simulink model "3DoFManipulatorWithBLDCM_SIMULATION"  (R2023b)
settings: Solver=VariableStepAuto  StartTime=0.0  StopTime=10  MaxStep=1e-4  RelTol=1e-3
undefined symbols (not defined in the file): X, Y, Z
libraries: spsMosfetLib x18, sm_lib x11, nesl_utility x7, eeGeneralControl x6, spsDCVoltageSourceLib x3, spsGroundLib x3, spsThreePhaseSeriesRLCBranchLib x3, spsThreePhaseVIMeasurementLib x3, slpidlib x3, sps_lib x1
(part 3 of 3)

== matlab function 3DoFManipulatorWithBLDCM_SIMULATION/BLDC/Actuator Link1/Three Phase Inverter/MOTOR_SPEED_BLOCK1 ==
  data: U_U input; U_V input; U_W input; U_U_PWM output; PWM input; U_V_PWM output; U_W_PWM output
function [U_U_PWM, U_V_PWM, U_W_PWM] = PWM_SPEED_BLOCK(U_U, U_V, U_W, PWM)
%#codegen

%    This function was generated by the Symbolic Math Toolbox version 23.2.
%    20-Mar-2024 19:58:52

U_U_PWM = 0;
U_V_PWM = 0;
U_W_PWM = 0;

% Apply PWM scaling based on input and PWM signal
if U_U ~= 0 && PWM ~= 0
    U_U_PWM = U_U * PWM;
end
if U_V ~= 0 && PWM ~= 0
    U_V_PWM = U_V * PWM;
end
if U_W ~= 0 && PWM ~= 0
    U_W_PWM = U_W * PWM;
end

end

== matlab function 3DoFManipulatorWithBLDCM_SIMULATION/BLDC/Actuator Link2/Three Phase Inverter/MOTOR_SPEED_BLOCK1 ==
  data: U_U input; U_V input; U_W input; U_U_PWM output; PWM input; U_V_PWM output; U_W_PWM output
function [U_U_PWM, U_V_PWM, U_W_PWM] = PWM_SPEED_BLOCK(U_U, U_V, U_W, PWM)
%#codegen

%    This function was generated by the Symbolic Math Toolbox version 23.2.
%    20-Mar-2024 19:58:52

U_U_PWM = 0;
U_V_PWM = 0;
U_W_PWM = 0;

% Apply PWM scaling based on input and PWM signal
if U_U ~= 0 && PWM ~= 0
    U_U_PWM = U_U * PWM;
end
if U_V ~= 0 && PWM ~= 0
    U_V_PWM = U_V * PWM;
end
if U_W ~= 0 && PWM ~= 0
    U_W_PWM = U_W * PWM;
end

end

== matlab function 3DoFManipulatorWithBLDCM_SIMULATION/Feedforward Control/PWM LINK1/MOTOR_SPEED_BLOCK3 ==
  data: e_diff input; dC output; p output
function [dC, p] = PWM_SPEED_BLOCK(e_diff)
%#codegen

%    This function was generated by the Symbolic Math Toolbox version 23.2.
%    20-Mar-2024 19:58:52

p = 0.0001;
p = max(1e-4, min(0.001, p));

% Sigmoidfunktion
dC = 1/(1+exp(-e_diff));
dC = max(0, min(0.99, dC));
end

== matlab function 3DoFManipulatorWithBLDCM_SIMULATION/Feedforward Control/PWM LINK2/MOTOR_SPEED_BLOCK3 ==
  data: e_diff input; dC output; p output
function [dC, p] = PWM_SPEED_BLOCK(e_diff)
%#codegen

%    This function was generated by the Symbolic Math Toolbox version 23.2.
%    20-Mar-2024 19:58:52

p = 0.0001;
p = max(1e-4, min(0.001, p));

% Sigmoidfunktion
dC = 1/(1+exp(-e_diff));
dC = max(0, min(0.99, dC));
end

== matlab function 3DoFManipulatorWithBLDCM_SIMULATION/Feedforward Control/PWM LINK2/diff_pos ==
  data: diff_pos output; t_pos input; t_vel input; a_pos input; CCW output
function [diff_pos, CCW] = differencePosition(t_pos, t_vel, a_pos)

if t_pos >= 0
    diff_pos = t_pos - a_pos;
    CCW = 0;
    if t_vel < 0
        diff_pos = (t_pos - a_pos)*(-1);
        CCW = 1;
    end
else
    diff_pos = (t_pos - a_pos)*(-1);
    CCW = 1;
    if t_vel > 0
        diff_pos = (t_pos - a_pos);
        CCW = 0;
    end
end

== matlab function 3DoFManipulatorWithBLDCM_SIMULATION/Feedforward Control/PWM LINK1/diff_pos ==
  data: diff_pos output; t_pos input; t_vel input; a_pos input; CCW output
function [diff_pos, CCW] = differencePosition(t_pos, t_vel, a_pos)

if t_pos >= 0
    diff_pos = t_pos - a_pos;
    CCW = 0;
    if t_vel < 0
        diff_pos = (t_pos - a_pos)*(-1);
        CCW = 1;
    end
else
    diff_pos = (t_pos - a_pos)*(-1);
    CCW = 1;
    if t_vel > 0
        diff_pos = (t_pos - a_pos);
        CCW = 0;
    end
end

== matlab function 3DoFManipulatorWithBLDCM_SIMULATION/BLDC/Actuator Link0/CURRENT_BLOCK ==
  data: I_U input; dI_U_OUT output; I_V input; U_U input; U_V input; U_W input; L input; R input; BEMF_U input; BEMF_V input; BEMF_W input; dI_V_OUT output; dI_W_OUT output
function [dI_U_OUT,dI_V_OUT,dI_W_OUT] = CURRENT_BLOCK(I_U,I_V,U_U,U_V,U_W,L,R,BEMF_U,BEMF_V,BEMF_W)
%#codegen

%    This function was generated by the Symbolic Math Toolbox version 23.2.
%    20-Mar-2024 19:08:31

% https://de.mathworks.com/matlabcentral/answers/446003-relation-between-flux-linkage-and-voltage-constant-power_pmsynchronousmachineparams
% based on the link the magnetic flux is approximately lamda
%LAMDA = (sqrt(2)/sqrt(3)) * ((48/sqrt(2))/P*W_M)
%LAMDA = 1/sqrt(3) * (K_T/1000*P) * (60/2*pi)

%U_UV = U_U - U_V;
%U_VW = U_V - U_W;

%dI_U_OUT = (U_UV.*2.0+U_VW-I_U.*R.*3.0+P*MFLUX*W_M*(-EMF_U.*2.0+EMF_V+EMF_W))./(L.*3.0);

%dI_V_OUT = (-U_UV+U_VW-I_V.*R.*3.0+P*MFLUX*W_M*(EMF_U-EMF_V.*2.0+EMF_W))./(L.*3.0);

%dI_W_OUT = -(dI_U_OUT+dI_V_OUT);

E_UW = BEMF_U - BEMF_W;
E_WV = BEMF_W - BEMF_V;

U_UW = U_U - U_W;
U_WV = U_W - U_V;

dI_U_OUT = (U_UW.*2.0 + U_WV - I_U.*R.*3.0 - E_UW.*2.0 - E_WV)./(L.*3.0);
dI_V_OUT = (-U_UW - U_WV.*2.0 - I_V.*R.*3.0 + E_UW + E_WV.*2.0)./(L.*3.0);
dI_W_OUT = -(dI_U_OUT+dI_V_OUT);

%dI_U_OUT = -(R*I_U)/L - (P*W_M*EMF_U)/(2*L) + U_U/L
%dI_V_OUT = -(R*I_V)/L - (P*W_M*EMF_V)/(2*L) + U_V/L
%dI_W_OUT = -(R*I_W)/L - (P*W_M*EMF_W)/(2*L) + U_W/L
%dI_W_OUT = -(dI_U_OUT+dI_V_OUT)
end

== matlab function 3DoFManipulatorWithBLDCM_SIMULATION/Feedforward Control/PWM LINK0/calculate duty cycle ==
  data: e_diff input; dC output; p output
function [dC, p] = PWM_DC_BLOCK(e_diff)
%#codegen

%    This function was generated by the Symbolic Math Toolbox version 23.2.
%    20-Mar-2024 19:58:52

p = 0.0001;
%p = max(1e-4, min(0.001, p));


% Sigmoidfunktion
dC = 1/(1+exp(-e_diff));
%dC = max(0, min(0.99, dC));
end

== matlab function 3DoFManipulatorWithBLDCM_SIMULATION/Feedforward Control/PWM LINK0/diff_pos ==
  data: diff_pos output; t_pos input; t_vel input; a_pos input; CCW output
function [diff_pos, CCW] = differencePosition(t_pos, t_vel, a_pos)

if t_pos >= 0
    diff_pos = t_pos - a_pos;
    CCW = 0;
    if t_vel < 0
        diff_pos = (t_pos - a_pos)*(-1);
        CCW = 1;
    end
else
    diff_pos = (t_pos - a_pos)*(-1);
    CCW = 1;
    if t_vel > 0
        diff_pos = (t_pos - a_pos);
        CCW = 0;
    end
end

== matlab function 3DoFManipulatorWithBLDCM_SIMULATION/Encoder/ENCODER_BLOCK_L0 ==
  data: encoder_output output; actual_position input
function encoder_output = simulateEncoder(actual_position)

    % https://www.siko-global.com/de-de/produkte/rotoline-drehgeber/absolute-drehgeber/wh5850
    % Auflösung wäre theoretisch 200pi/2^19
    resolution = 0.0012;
    delay = 0.0001;
    dt = 2e-4;

    % quantizes
    quantized_position = round(actual_position / resolution) * resolution;

    % delay
    persistent position_queue;
    if isempty(position_queue)
        position_queue = repmat(quantized_position, 1, round(delay/dt));
    end
    encoder_output = position_queue(1)/100;
    position_queue = [position_queue(2:end), quantized_position];
    
end

== matlab function 3DoFManipulatorWithBLDCM_SIMULATION/Feedforward Control/INVERSE_DYNAMICS_BLOCK ==
  data: b0 input; tau0 output; b1 input; b2 input; ddq0 input; ddq1 input; ddq2 input; dq0 input; dq1 input; dq2 input; g input; l1 input; l2 input; m0 input; m1 input; m2 input; q1 input; q2 input; r0 input; r1 input; r2 input; tau1 output; tau2 output
function [tau0,tau1,tau2] = INVERSE_DYNAMICS_BLOCK(b0,b1,b2,ddq0,ddq1,ddq2,dq0,dq1,dq2,g,l1,l2,m0,m1,m2,q1,q2,r0,r1,r2)
%#codegen

%    This function was generated by the Symbolic Math Toolbox version 23.2.
%    20-Feb-2024 15:14:27

% b0 = complex(b0);  % if required to enforce complex operations
% b1 = complex(b1);  % if required to enforce complex operations
% b2 = complex(b2);  % if required to enforce complex operations
% ddq0 = complex(ddq0);  % if required to enforce complex operations
% ddq1 = complex(ddq1);  % if required to enforce complex operations
% ddq2 = complex(ddq2);  % if required to enforce complex operations
% dq0 = complex(dq0);  % if required to enforce complex operations
% dq1 = complex(dq1);  % if required to enforce complex operations
% dq2 = complex(dq2);  % if required to enforce complex operations
% g = complex(g);  % if required to enforce complex operations
% l1 = complex(l1);  % if required to enforce complex operations
% l2 = complex(l2);  % if required to enforce complex operations
% m0 = complex(m0);  % if required to enforce complex operations
% m1 = complex(m1);  % if required to enforce complex operations
% m2 = complex(m2);  % if required to enforce complex operations
% q1 = complex(q1);  % if required to enforce complex operations
% q2 = complex(q2);  % if required to enforce complex operations
% r0 = complex(r0);  % if required to enforce complex operations
% r1 = complex(r1);  % if required to enforce complex operations
% r2 = complex(r2);  % if required to enforce complex operations
et1 = b0.*dq0+(ddq0.*m0.*r0.^2)./2.0+ddq0.*m1.*r1.^2.*(3.0./8.0)+ddq0.*m2.*r2.^2.*(3.0./8.0)+(ddq0.*l1.^2.*m1)./6.0+(ddq0.*l1.^2.*m2)./2.0+(ddq0.*l2.^2.*m2)./6.0+(ddq0.*l1.^2.*m1.*cos(q1.*2.0))./1.2e+1+(ddq0.*l1.^2.*m2.*cos(q1.*2.0))./2.0+(ddq0.*m1.*r1.^2.*cos(q1.*2.0))./8.0+(ddq0.*l2.^2.*m2.*cos(q1.*2.0+q2.*2.0))./1.2e+1+(ddq0.*m2.*r2.^2.*cos(q1.*2.0+q2.*2.0))./8.0+(ddq0.*l1.*l2.*m2.*cos(q1.*2.0+q2))./2.0-(dq0.*dq1.*l1.^2.*m1.*sin(q1.*2.0))./6.0-dq0.*dq1.*l1.^2.*m2.*sin(q1.*2.0)-(dq0.*dq1.*m1.*r1.^2.*sin(q1.*2.0))./4.0;
et2 = dq0.*dq1.*l2.^2.*m2.*sin(q1.*2.0+q2.*2.0).*(-1.0./6.0)-(dq0.*dq2.*l2.^2.*m2.*sin(q1.*2.0+q2.*2.0))./6.0-(dq0.*dq1.*m2.*r2.^2.*sin(q1.*2.0+q2.*2.0))./4.0-(dq0.*dq2.*m2.*r2.^2.*sin(q1.*2.0+q2.*2.0))./4.0+(ddq0.*l1.*l2.*m2.*cos(q2))./2.0-(dq0.*dq2.*l1.*l2.*m2.*sin(q2))./2.0-dq0.*dq1.*l1.*l2.*m2.*sin(q1.*2.0+q2)-(dq0.*dq2.*l1.*l2.*m2.*sin(q1.*2.0+q2))./2.0;
tau0 = et1+et2;
if nargout > 1
    et3 = b1.*dq1+(ddq1.*m1.*r1.^2)./4.0+(ddq1.*m2.*r2.^2)./4.0+(ddq2.*m2.*r2.^2)./4.0+(ddq1.*l1.^2.*m1)./3.0+ddq1.*l1.^2.*m2+(ddq1.*l2.^2.*m2)./3.0+(ddq2.*l2.^2.*m2)./3.0+(g.*l2.*m2.*cos(q1+q2))./2.0+(g.*l1.*m1.*cos(q1))./2.0+g.*l1.*m2.*cos(q1)+(dq0.^2.*l1.^2.*m1.*sin(q1.*2.0))./1.2e+1+(dq0.^2.*l1.^2.*m2.*sin(q1.*2.0))./2.0+(dq0.^2.*m1.*r1.^2.*sin(q1.*2.0))./8.0+(dq0.^2.*l2.^2.*m2.*sin(q1.*2.0+q2.*2.0))./1.2e+1+(dq0.^2.*m2.*r2.^2.*sin(q1.*2.0+q2.*2.0))./8.0-(dq2.^2.*l1.*l2.*m2.*sin(q2))./2.0;
    et4 = (dq0.^2.*l1.*l2.*m2.*sin(q1.*2.0+q2))./2.0+ddq1.*l1.*l2.*m2.*cos(q2)+(ddq2.*l1.*l2.*m2.*cos(q2))./2.0-dq1.*dq2.*l1.*l2.*m2.*sin(q2);
    tau1 = et3+et4;
end
if nargout > 2
    tau2 = b2.*dq2+(ddq1.*m2.*r2.^2)./4.0+(ddq2.*m2.*r2.^2)./4.0+(ddq1.*l2.^2.*m2)./3.0+(ddq2.*l2.^2.*m2)./3.0+(g.*l2.*m2.*cos(q1+q2))./2.0+(dq0.^2.*l2.^2.*m2.*sin(q1.*2.0+q2.*2.0))./1.2e+1+(dq0.^2.*m2.*r2.^2.*sin(q1.*2.0+q2.*2.0))./8.0+(dq0.^2.*l1.*l2.*m2.*sin(q2))./4.0+(dq1.^2.*l1.*l2.*m2.*sin(q2))./2.0+(dq0.^2.*l1.*l2.*m2.*sin(q1.*2.0+q2))./4.0+(ddq1.*l1.*l2.*m2.*cos(q2))./2.0;
end
end

== matlab function 3DoFManipulatorWithBLDCM_SIMULATION/BLDC/Actuator Link0/BACK_EMF_BLOCK ==
  data: W_M input; K_E input; THETA_E input; BEMF_U output; BEMF_V output; BEMF_W output
function [BEMF_U, BEMF_V, BEMF_W] = BEMF_BLOCK(W_M, K_E, THETA_E)
%#codegen

%    This function was generated by the Symbolic Math Toolbox version 23.2.
%    20-Mar-2024 19:08:31

%THETA = mod(THETA_E,  2*pi);
THETA = THETA_E;
% electrical theta 0°-60°
if (0 <= THETA) && (THETA < 1*pi/3)
    F_U = 1;
    F_V = -1;
    F_W = 1-6*THETA/pi;

% electrical theta 60°-120°
elseif (1*pi/3 <= THETA) &&(THETA < 2*pi/3)
    F_U = 1;
    F_V = 6*THETA/pi - 3;
    F_W = -1;

% electrical theta 120°-180°
elseif (2*pi/3 <= THETA) && (THETA < pi)
    F_U = -6*THETA/pi + 5;
    F_V = 1;
    F_W = -1;

% electrical theta 180°-240°
elseif (pi <= THETA) && (THETA < 4*pi/3)
    F_U = -1;
    F_V = 1;
    F_W = 6*THETA/pi -7;

% electrical theta 240°-300°
elseif (4*pi/3 <= THETA) && (THETA < 5*pi/3)
    F_U = -1;
    F_V = -6*THETA/pi + 9;
    F_W = 1;

% electrical theta 300°-360°
elseif (5*pi/3 <= THETA) && (THETA < 2*pi)
    F_U = 6*THETA/pi - 11;
    F_V = -1;
    F_W = 1;

% something went wrong
else
    F_U = NaN;
    F_V = NaN;
    F_W = NaN;
end

BEMF_U = K_E*W_M*F_U;
BEMF_V = K_E*W_M*F_V;
BEMF_W = K_E*W_M*F_W;

end

== matlab function 3DoFManipulatorWithBLDCM_SIMULATION/BLDC/Actuator Link0/ROTOR_SPEED_BLOCK/TO_THETAE_BLOCK ==
  data: theta output; theta input
function theta = generateTheta(theta)
    theta = mod(theta, 2*pi);
end
